simulink subsystem "subsyssesnores"  (R2023b)
settings: Solver=VariableStepAuto  StartTime=0.0  StopTime=10.0  RelTol=1e-3
libraries: arduinolib x2
settings Model: Creator=Usuario_UMA  LastModifiedBy=Usuario_UMA

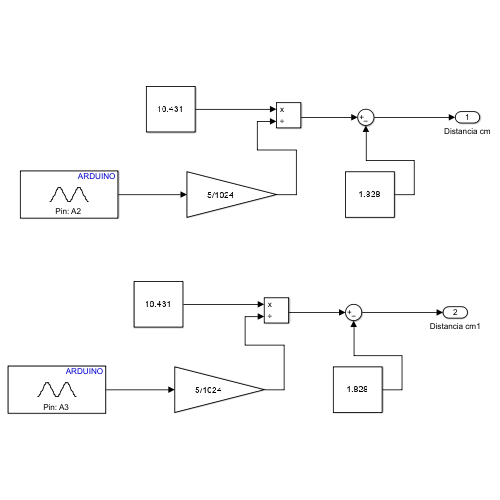
[thumbnail: Simulink's stored preview of the top-level diagram]
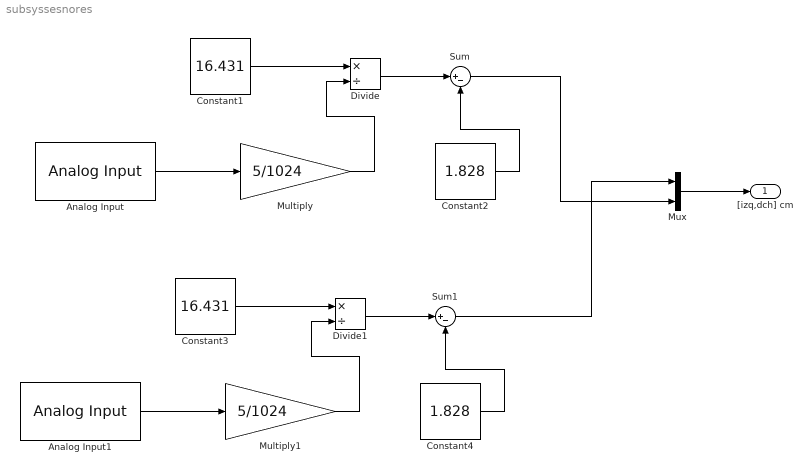
== system subsyssesnores ==
  Analog Input : arduinolib/Analog Input  pinNumber=2  ReadResultsOnly=off  ConversionTriggerSource=Software  ExternalTriggerType=uint32( 0 )  OutputDataType=uint16  EnableConversionCompleteNotify=off  EnableOuputStatus=off  SampleTime=-1  blockPlatform=arduino
  Analog Input1 : arduinolib/Analog Input  pinNumber=3  ReadResultsOnly=off  ConversionTriggerSource=Software  ExternalTriggerType=uint32( 0 )  OutputDataType=uint16  EnableConversionCompleteNotify=off  EnableOuputStatus=off  SampleTime=-1  blockPlatform=arduino
  Constant1 : Constant  Value=16.431
  Constant2 : Constant  Value=1.828
  Constant3 : Constant  Value=16.431
  Constant4 : Constant  Value=1.828
  Divide : Product  Inputs=*/
  Divide1 : Product  Inputs=*/
  Multiply : Gain  Gain=5/1024
  Multiply1 : Gain  Gain=5/1024
  Mux : Mux  Inputs=2
  Sum : Sum  Inputs=|+-
  Sum1 : Sum  Inputs=|+-
  "[izq,dch] cm" : Outport
  wires:
  Multiply1/1 -> Divide1/2
  Multiply/1 -> Divide/2
  Analog Input/1 -> Multiply/1
  Constant1/1 -> Divide/1
  Constant3/1 -> Divide1/1
  Analog Input1/1 -> Multiply1/1
  Constant4/1 -> Sum1/2
  Divide1/1 -> Sum1/1
  Constant2/1 -> Sum/2
  Divide/1 -> Sum/1
  Mux/1 -> "[izq,dch] cm"/1
  Sum/1 -> Mux/2
  Sum1/1 -> Mux/1
